simulink model "ex_kalman22"  (R2017a)
settings: Solver=FixedStepDiscrete  StartTime=0.0  StopTime=61  RelTol=1e-3  EnableMultiTasking=on
InitFcn:
  | load position.mat;
  | [R,C]=size(position);
  | FRAME_SIZE=5;
  | idx=(1:FRAME_SIZE:C)';
  | LEN=length(idx);
  | t=(1:LEN)'-1;
undefined symbols (not defined in the file or in its folder): position
settings Model: Creator=The MathWorks, Inc.  LastModifiedBy=The MathWorks, Inc.
settings DataIOCC: LimitDataPoints=on  SaveFormat=Array
settings OptimizationCC: ExpressionDepthLimit=2147483647  LifeSpan=inf
settings DebuggingCC: UnderspecifiedInitializationDetection=Classic  MergeDetectMultiDrivingBlocksExec=none  SolverPrmCheckMsg=warning  FcnCallInpInsideContextMsg=warning  StateNameClashWarn=warning  SFUnexpectedBacktrackingDiag=warning  SFNoUnconditionalDefaultTransitionDiag=warning  SFExecutionAtInitializationDiag=none
settings HardwareCC: ProdBitPerPointer=32  ProdBitPerSizeT=32  ProdBitPerPtrDiffT=32  ProdLargestAtomicFloat=None  ProdIntDivRoundTo=Undefined  ProdEndianess=Unspecified  ProdWordSize=32  ProdHWDeviceType=32-bit Generic
settings ModelReferenceCC: PropagateSignalLabelsOutOfModel=off
settings SFSimCC: SimParseCustomCode=off
settings GRTTargetCC: TargetLangStandard=C89/C90 (ANSI)  GeneratePreprocessorConditionals=Disable all  CombineOutputUpdateFcns=off  GRTInterface=on
settings ConfigComp: CovMetricSettings=dw  CovHtmlReporting=on  CovSaveCumulativeToWorkspaceVar=on  CovSaveSingleToWorkspaceVar=on  CovExternalEMLEnable=off

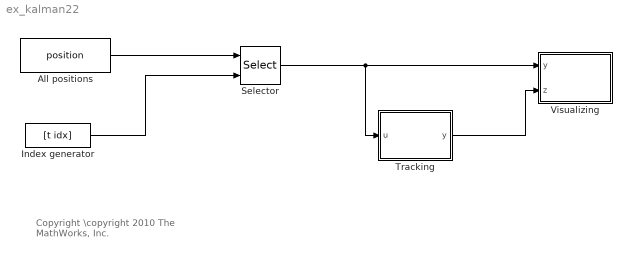
== system ex_kalman22 ==
  note: Copyright \copyright 2010 The MathWorks, Inc.
  "    Index generator" : FromWorkspace  VariableName=[t idx]  SampleTime=1  Interpolate=off  OutputAfterFinalValue=Holding final value
  All positions : Constant  Value=position
  Selector : Selector  NumberOfDimensions=2  InputPortWidth=2  IndexOptions=Select all,Starting index (port)  Indices=[1 3],2  OutputSizes=1,FRAME_SIZE
  Tracking : MATLAB Function  TreatAsAtomicUnit=on
  Visualizing : MATLAB Function  TreatAsAtomicUnit=on
  wires:
  Selector/1 -> Tracking/1(u), Visualizing/1(y)
  Tracking/1(y) -> Visualizing/2(z)
  All positions/1 -> Selector/1
  "    Index generator"/1 -> Selector/2

== matlab function ex_kalman22/Visualizing ==
  data: y input; z input
function plot_me(y,z)
%#codegen
coder.extrinsic('figure','hold','plot_trajectory');
persistent h
if isempty(h)
  h=figure;
  hold;
end
plot_trajectory(y,z);
end

== matlab function ex_kalman22/Tracking ==
  data: u input; y output
function y = kalman(u)
%#codegen

y = ex_kalman03(u);
